simulink model "PD_Controller_RigidJoint"  (R2019b)
settings: Solver=VariableStepAuto  StartTime=0.0  StopTime=10  RelTol=1e-3
libraries: simulink x2, robotcorelib x1
settings Model: Creator=USER  LastModifiedBy=USER

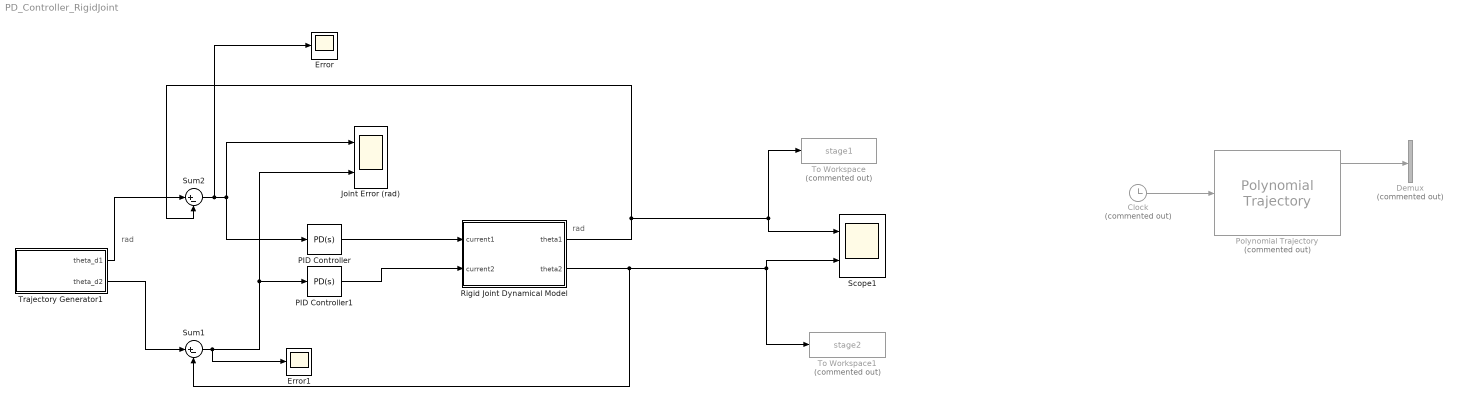
== system PD_Controller_RigidJoint ==
  note: rad
  note: rad
  Clock : Clock  Commented=on
  Demux : Demux  Commented=on  Outputs=2
  Error : Scope
  Error1 : Scope
  Joint Error (rad) : Scope  NumInputPorts=2
  PID Controller : simulink/Continuous/PID Controller  Controller=PD  Form=Parallel  TimeDomain=Continuous-time  SampleTime=-1  IntegratorMethod=Forward Euler  FilterMethod=Forward Euler  ControllerParametersSource=internal  P=3  I=0.00248207984793386  D=0.6  UseFilter=on  N=100  TunerSelectOption=Transfer Function Based (PID Tuner App)  InitialConditionSource=internal  InitialConditionForIntegrator=0  InitialConditionForFilter=0  DifferentiatorICPrevScaledInput=0  ExternalReset=none  TrackingMode=off  Kt=1  LimitOutput=off  UpperSaturationLimit=inf  LowerSaturationLimit=-inf  LinearizeAsGain=on  AntiWindupMode=none  Kb=1  POutMin=[]  POutMax=[]  IOutMin=[]  IOutMax=[]  DOutMin=[]  DOutMax=[]  NOutMin=[]  NOutMax=[]  SumOutMin=[]  SumOutMax=[]  SaturationOutMin=[]  SaturationOutMax=[]  PParamMin=[]  PParamMax=[]  IParamMin=[]  IParamMax=[]  DParamMin=[]  DParamMax=[]  NParamMin=[]  NParamMax=[]  KbParamMin=[]  KbParamMax=[]  KtParamMin=[]  KtParamMax=[]  KbOutMin=[]  KbOutMax=[]  KtOutMin=[]  KtOutMax=[]  IntegratorOutMin=[]  IntegratorOutMax=[]  FilterOutMin=[]  FilterOutMax=[]  SumI1OutMin=[]  SumI1OutMax=[]  SumI2OutMin=[]  SumI2OutMax=[]  SumI3OutMin=[]  SumI3OutMax=[]  SumI4OutMin=[]  SumI4OutMax=[]  SumDOutMin=[]  SumDOutMax=[]  DifferentiatorOutMin=[]  DifferentiatorOutMax=[]  FilterDiffOutCoefMin=[]  FilterDiffOutCoefMax=[]  ReciprocalOutMin=[]  ReciprocalOutMax=[]  SumDenOutMin=[]  SumDenOutMax=[]  SumNumOutMin=[]  SumNumOutMax=[]  DivideOutMin=[]  DivideOutMax=[]  IntegratorContinuousStateAttributes=''  IntegratorStateMustResolveToSignalObject=off  IntegratorRTWStateStorageClass=Auto  FilterContinuousStateAttributes=''  FilterStateMustResolveToSignalObject=off  FilterRTWStateStorageClass=Auto  ParallelPVariant=InternalParameters  IdealPVariant=Disabled  IVariant=Disabled  DVariant=InternalParameters  IntegratorVariant=Disabled  SatVariant=Disabled  AWVariant=Disabled  PCopyVariant=Disabled  TRVariant=Disabled  FdbkBlocksVariant=Forward  IdealPFdbkVariant=Disabled  SatFdbkVariant=Disabled  DerivativeFilterVariant=ContFilter  NVariant=InternalParameters  NCopyVariant=Disabled  FilterICVariant=InternalICsFilter  IntegratorICVariant=Disabled  ExternalResetVariant=Disabled  TRSumVariant=Passthrough  SumFdbkVariant=Disabled  SumVariant=Sum_PD
  PID Controller1 : simulink/Continuous/PID Controller  Controller=PD  Form=Parallel  TimeDomain=Continuous-time  SampleTime=-1  IntegratorMethod=Forward Euler  FilterMethod=Forward Euler  ControllerParametersSource=internal  P=3  I=0.00248207984793386  D=0.5  UseFilter=on  N=100  TunerSelectOption=Transfer Function Based (PID Tuner App)  InitialConditionSource=internal  InitialConditionForIntegrator=0  InitialConditionForFilter=0  DifferentiatorICPrevScaledInput=0  ExternalReset=none  TrackingMode=off  Kt=1  LimitOutput=off  UpperSaturationLimit=inf  LowerSaturationLimit=-inf  LinearizeAsGain=on  AntiWindupMode=none  Kb=1  POutMin=[]  POutMax=[]  IOutMin=[]  IOutMax=[]  DOutMin=[]  DOutMax=[]  NOutMin=[]  NOutMax=[]  SumOutMin=[]  SumOutMax=[]  SaturationOutMin=[]  SaturationOutMax=[]  PParamMin=[]  PParamMax=[]  IParamMin=[]  IParamMax=[]  DParamMin=[]  DParamMax=[]  NParamMin=[]  NParamMax=[]  KbParamMin=[]  KbParamMax=[]  KtParamMin=[]  KtParamMax=[]  KbOutMin=[]  KbOutMax=[]  KtOutMin=[]  KtOutMax=[]  IntegratorOutMin=[]  IntegratorOutMax=[]  FilterOutMin=[]  FilterOutMax=[]  SumI1OutMin=[]  SumI1OutMax=[]  SumI2OutMin=[]  SumI2OutMax=[]  SumI3OutMin=[]  SumI3OutMax=[]  SumI4OutMin=[]  SumI4OutMax=[]  SumDOutMin=[]  SumDOutMax=[]  DifferentiatorOutMin=[]  DifferentiatorOutMax=[]  FilterDiffOutCoefMin=[]  FilterDiffOutCoefMax=[]  ReciprocalOutMin=[]  ReciprocalOutMax=[]  SumDenOutMin=[]  SumDenOutMax=[]  SumNumOutMin=[]  SumNumOutMax=[]  DivideOutMin=[]  DivideOutMax=[]  IntegratorContinuousStateAttributes=''  IntegratorStateMustResolveToSignalObject=off  IntegratorRTWStateStorageClass=Auto  FilterContinuousStateAttributes=''  FilterStateMustResolveToSignalObject=off  FilterRTWStateStorageClass=Auto  ParallelPVariant=InternalParameters  IdealPVariant=Disabled  IVariant=Disabled  DVariant=InternalParameters  IntegratorVariant=Disabled  SatVariant=Disabled  AWVariant=Disabled  PCopyVariant=Disabled  TRVariant=Disabled  FdbkBlocksVariant=Forward  IdealPFdbkVariant=Disabled  SatFdbkVariant=Disabled  DerivativeFilterVariant=ContFilter  NVariant=InternalParameters  NCopyVariant=Disabled  FilterICVariant=InternalICsFilter  IntegratorICVariant=Disabled  ExternalResetVariant=Disabled  TRSumVariant=Passthrough  SumFdbkVariant=Disabled  SumVariant=Sum_PD
  Polynomial Trajectory : robotcorelib/Polynomial Trajectory  Commented=on  WaypointSource=Internal  Waypoints=[ 0, deg2rad(15), deg2rad(30), deg2rad(45), deg2rad(60); 0 deg2rad(30), deg2rad(60), deg2rad(90), deg2rad(60) ]  TimePoints=[ 0, 4, 8, 12, 16 ]  TimeInterval=[ 1, 4 ]  Method=Cubic Polynomial  ParameterSource=Internal  VelocityBoundaryCondition=zeros( 2, 5 )  AccelerationBoundaryCondition=zeros( 2, 5 )  SimulateUsing=Interpreted execution
      settings: SourceProductName=Robotics System Toolbox  SourceProductBaseCode=RO
  Rigid Joint Dynamical Model : Subsystem
  Scope1 : Scope  NumInputPorts=2
  Sum1 : Sum  Inputs=|+-
  Sum2 : Sum  Inputs=|+-
  To Workspace : ToWorkspace  Commented=on  VariableName=stage1  SaveFormat=Timeseries  SampleTime=-1
  To Workspace1 : ToWorkspace  Commented=on  VariableName=stage2  SaveFormat=Timeseries  SampleTime=-1
  Trajectory Generator1 : MATLAB Function  TreatAsAtomicUnit=on
  wires:
  PID Controller/1 -> Rigid Joint Dynamical Model/1(current1)
  Trajectory Generator1/1(theta_d1) -> Sum2/1
  PID Controller1/1 -> Rigid Joint Dynamical Model/2("current2 ")
  Rigid Joint Dynamical Model/2(theta2) -> To Workspace1/1, Scope1/2, Sum1/2
  Rigid Joint Dynamical Model/1(theta1) -> Scope1/1, To Workspace/1, Sum2/2
  Sum2/1 -> Error/1, Joint Error (rad)/1, PID Controller/1
  Sum1/1 -> Error1/1, Joint Error (rad)/2, PID Controller1/1
  Trajectory Generator1/2(theta_d2) -> Sum1/1
  Polynomial Trajectory/1 -> Demux/1
  Clock/1 -> Polynomial Trajectory/1

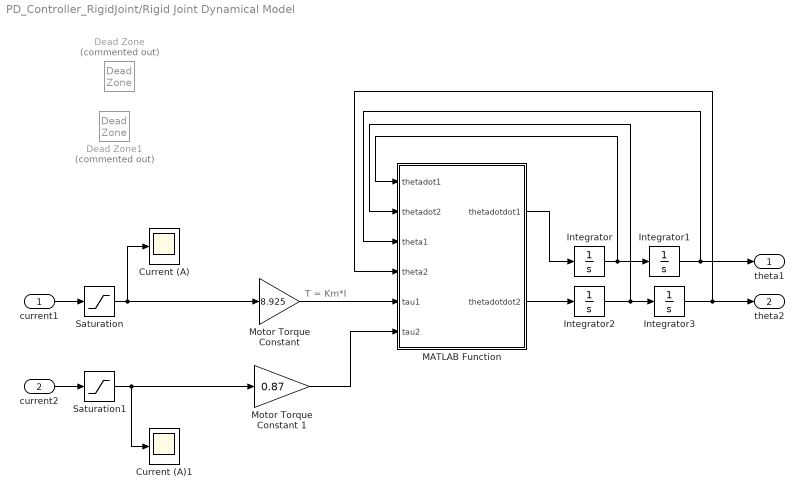
== system PD_Controller_RigidJoint/Rigid Joint Dynamical Model ==
  note: T = Km*I
  current1 : Inport
  "current2 " : Inport  Port=2
  Current (A) : Scope
  Current (A)1 : Scope
  Dead Zone : DeadZone  Commented=on  LowerValue=-0.2  UpperValue=0.2  SaturateOnIntegerOverflow=on
  Dead Zone1 : DeadZone  Commented=on  LowerValue=-0.15  UpperValue=0.15  SaturateOnIntegerOverflow=on
  Integrator{,1..3} (4 alike) : Integrator
  MATLAB Function : MATLAB Function  TreatAsAtomicUnit=on
  "Motor Torque Constant " : Gain  Gain=8.925
  Motor Torque Constant 1 : Gain  Gain=0.87
  Saturation : Saturate  UpperLimit=1  LowerLimit=-1
  Saturation1 : Saturate
  theta1 : Outport
  theta2 : Outport  Port=2
  wires:
  Integrator1/1 -> MATLAB Function/3(theta1), theta1/1
  "Motor Torque Constant "/1 -> MATLAB Function/5(tau1)
  Integrator/1 -> MATLAB Function/1(thetadot1), Integrator1/1
  MATLAB Function/1(thetadotdot1) -> Integrator/1
  current1/1 -> Saturation/1
  MATLAB Function/2(thetadotdot2) -> Integrator2/1
  Integrator2/1 -> MATLAB Function/2(thetadot2), Integrator3/1
  Integrator3/1 -> MATLAB Function/4(theta2), theta2/1
  Motor Torque Constant 1/1 -> MATLAB Function/6(tau2)
  "current2 "/1 -> Saturation1/1
  Saturation/1 -> "Motor Torque Constant "/1, Current (A)/1
  Saturation1/1 -> Motor Torque Constant 1/1, Current (A)1/1

== matlab function PD_Controller_RigidJoint/Trajectory Generator1 ==
  data: theta_d1 output; theta_d2 output
function [theta_d1,theta_d2]  = fcn
theta_start1 = 0;
theta_start2 = 0;
theta_end1 = pi/4;
theta_end2 = pi/4;
theta_d1 = theta_start1 + (theta_end1-theta_start1);
theta_d2 = theta_start2 + (theta_end2-theta_start2);

== matlab function PD_Controller_RigidJoint/Rigid Joint Dynamical Model/MATLAB Function ==
  data: thetadot1 input; thetadotdot1 output; thetadot2 input; theta1 input; theta2 input; tau1 input; thetadotdot2 output; tau2 input
function [thetadotdot1,thetadotdot2] = fcn(thetadot1,thetadot2,theta1,theta2,tau1,tau2)
%y is thetadotdot
tau = [tau1;tau2];
%Veltman Thesis Values
% m1 = 0.5; 
% m2 = 1;
% L1 = 0.343;
% L2 = 0.267;
% Lc1 = 0.2;
% Lc2 = 0.25;
% I1 = 0.01;
% I2 = 0.01;
% B1 = 0.070364;
% B2 = 0.028211;

%Electrical School values
m1 =  1.51 ; 
m2 = 0.87326;
L1 = 0.343;
L2 = 0.267;
Lc1 = 0.1590;
Lc2 = 0.0550;
I1 = 0.0392;
I2 = 0.0081;
B1 = 0.070364;
B2 = 0.028211;


M11 = I2+I1+m2*((L1^2)+(Lc2^2)+2*L1*Lc2*cos(theta2))+m1*(Lc1^2);
M12 = I2+m2*(Lc2^2)+L1*Lc2*m2*cos(theta2);
M21 = M12;
M22 = I2+m2*(Lc2^2);

M = [M11 M12;
     M21 M22];
 
C11 = -m2*L1*Lc2*sin(theta2)*thetadot2;
C12 = -m2*L1*Lc2*sin(theta2)*thetadot2-m2*L1*Lc2*sin(theta2)*thetadot1;
C21 = m2*L1*Lc2*sin(theta2)*thetadot1;
C22 = 0;

C = [C11 C12;
     C21 C22];

C1 = C*[thetadot1;thetadot2];
 
fv = [B1 0;0 B2]*[thetadot1;thetadot2];

thetadotdot = inv(M)*(tau-C1-fv);
thetadotdot1 = thetadotdot(1);
thetadotdot2 = thetadotdot(2);
